simulink model "IM"  (R2017a)
settings: Solver=VariableStepAuto  StartTime=0.0  StopTime=simpletime  RelTol=1e-3
values from neighbouring files (symbols this model uses):
  dt = 0.1    [exmM_IM.m]
settings Model: Creator=lzr96  LastModifiedBy=lzr96

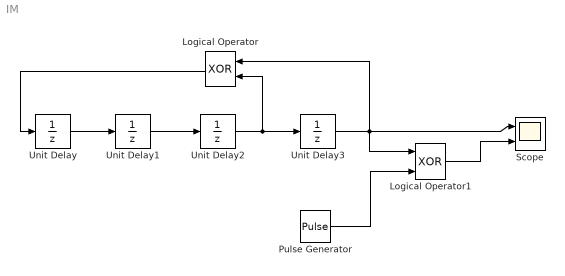
== system IM ==
  Logical Operator : Logic  Operator=XOR  AllPortsSameDT=off  OutDataTypeStr=boolean
  Logical Operator1 : Logic  Operator=XOR  AllPortsSameDT=off  OutDataTypeStr=boolean
  Pulse Generator : DiscretePulseGenerator  PulseType=Time based  Period=dt*2  PulseWidth=50
  Scope : Scope  NumInputPorts=2
  Unit Delay : UnitDelay  InitialCondition=1  SampleTime=-1
  Unit Delay1 : UnitDelay  SampleTime=-1
  Unit Delay2 : UnitDelay  SampleTime=-1
  Unit Delay3 : UnitDelay  SampleTime=-1
  wires:
  Logical Operator/1 -> Unit Delay/1
  Unit Delay3/1 -> Scope/1, Logical Operator/1, Logical Operator1/1
  Unit Delay1/1 -> Unit Delay2/1
  Unit Delay/1 -> Unit Delay1/1
  Unit Delay2/1 -> Logical Operator/2, Unit Delay3/1
  Pulse Generator/1 -> Logical Operator1/2
  Logical Operator1/1 -> Scope/2
